simulink model "fourthslx"  (R2022a)
settings: Solver=VariableStepAuto  StartTime=0.0  StopTime=10.0  RelTol=1e-3
undefined symbols (not defined in the file): doppler, pskmod
libraries: commdigbbndpm3 x2, commsink2 x1, commeq3 x1, commrandsrc3 x1, commchan3 x1
settings Model: Creator=Admin  LastModifiedBy=Admin

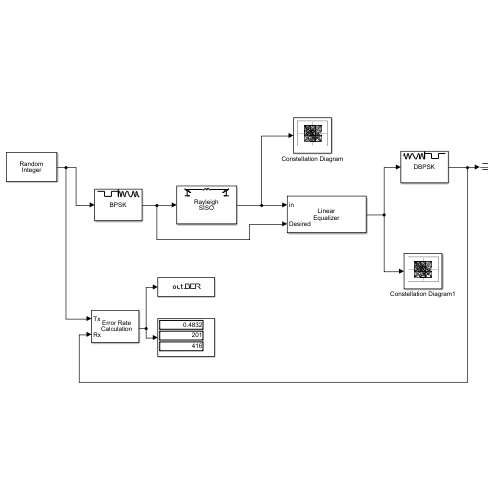
[thumbnail: Simulink's stored preview of the top-level diagram]
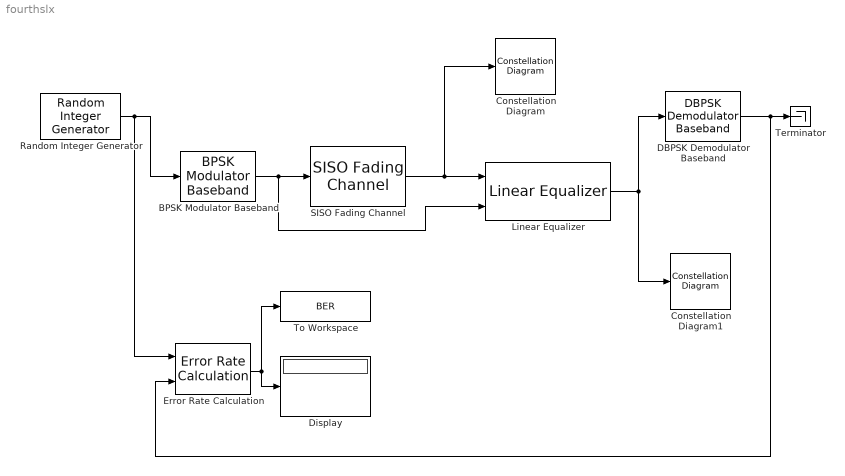
== system fourthslx ==
  BPSK Modulator Baseband : commdigbbndpm3/BPSK Modulator Baseband  Ph=0  outDtype=double  outWordLen=16  outUDDataType=sfix(16)  outFracLenMode=Best precision  outFracLen=15  outDataTypeStr=double  outLastDataTypeStr=double
  Constellation Diagram : ConstellationDiagram  WindowPosition=[382.000000,84.000000,600.000000,600.000000,]  ScopeFrameLocation=window  ShowTrajectory=on
  Constellation Diagram1 : ConstellationDiagram  WindowPosition=[146.000000,105.000000,600.000000,600.000000,]  ScopeFrameLocation=window  ReferenceConstellation="[0.70711+0.70711i        -0.70711+0.70711i        -0.70711-0.70711i         0.70711-0.70711i]"  XLimits=[-1.46,1.46]  YLimits=[-1.38,1.38]  ShowTrajectory=on  EnableMeasurements=on
  DBPSK Demodulator Baseband : commdigbbndpm3/DBPSK Demodulator Baseband  Ph=0  outDtype=Inherit via internal rule
      settings: SourceProductBaseCode=CM
  Display : Display
  Error Rate Calculation : commsink2/Error Rate Calculation  N=0  st_delay=0  cp_mode=Entire frame  subframe=[]  PMode=Port  WsName=ErrorVec  RsMode2=off  stop=on  numErr=200  maxBits=500
  Linear Equalizer : commeq3/Linear Equalizer  NumTaps=4  Constellation=pskmod( 0:1, 2, pi/4, 'bin' )  InputSamplesPerSymbol=1  Algorithm=LMS  StepSize=0.1  ForgettingFactor=0.99  InitialInverseCorrelationMatrix=0.1  ReferenceTap=2  InputDelay=0  AdaptWeightsSource=Property  AdaptWeights=on  InitialWeightsSource=Auto  InitialWeights=0  TrainingInitialWeights=0  BlindInitialWeights=[ 0; 0; 1; 0; 0 ]  WeightUpdatePeriod=1  TrainingFlagInputPort=off  AdaptAfterTraining=on  ResetInputPort=off  ErrorOutputPort=off  TapWeightsOutputPort=off  SimulateUsing=Code generation
      settings: SourceProductBaseCode=CM
  Random Integer Generator : commrandsrc3/Random Integer Generator  SetSize=2  SeedSource=Auto  Seed=0  SampleTime=1/500000  SamplesPerFrame=8  OutputDataType=double  SimulateUsing=Interpreted execution
  SISO Fading Channel : commchan3/SISO Fading Channel  InheritSampleRate=on  SampleRate=1  PathDelays=2.24  AveragePathGains=9  NormalizePathGains=on  FadingDistribution=Rayleigh  KFactor=3  DirectPathDopplerShift=0  DirectPathInitialPhase=0  MaximumDopplerShift=100  DopplerSpectrum=doppler('Jakes')  RandomStream=mt19937ar with seed  Seed=73  PathGainsOutputPort=off  ChannelFilterDelayOutputPort=off  SimulateUsing=Interpreted execution  Visualization=Off  PathsForDopplerDisplay=1  SamplesToDisplay=25%
  Terminator : Terminator
  To Workspace : ToWorkspace  VariableName=BER  SaveFormat=Timeseries  SampleTime=-1
  wires:
  Random Integer Generator/1 -> Error Rate Calculation/1, BPSK Modulator Baseband/1
  BPSK Modulator Baseband/1 -> Linear Equalizer/2, SISO Fading Channel/1
  Error Rate Calculation/1 -> To Workspace/1, Display/1
  SISO Fading Channel/1 -> Constellation Diagram/1, Linear Equalizer/1
  Linear Equalizer/1 -> DBPSK Demodulator Baseband/1, Constellation Diagram1/1
  DBPSK Demodulator Baseband/1 -> Error Rate Calculation/2, Terminator/1
